simulink model "WT_MPPT_SCOPES_FINAL_v3"  (R2025a)
settings: Solver=ode4  StartTime=0.0  StopTime=11  FixedStep=0.1  RelTol=1e-3
settings Model: Creator=hero  LastModifiedBy=hero

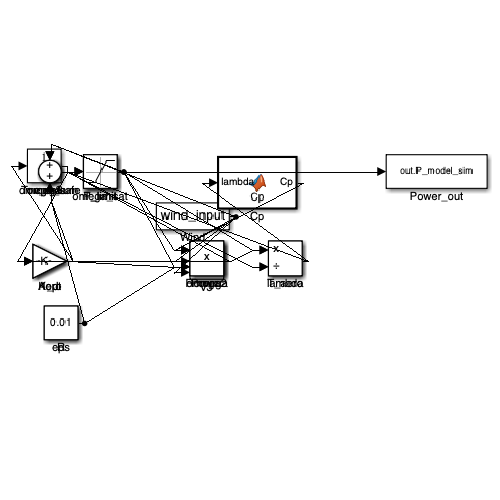
[thumbnail: Simulink's stored preview of the top-level diagram]
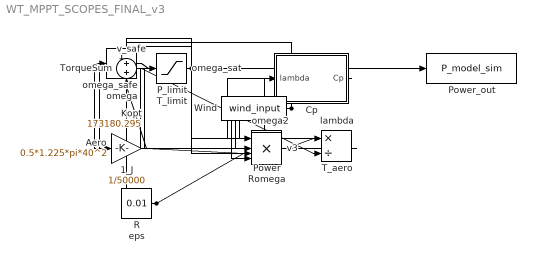
== system WT_MPPT_SCOPES_FINAL_v3 ==
  1_J : Gain  Gain=1/50000
  Aero : Gain  Gain=0.5*1.225*pi*40^2
  Cp : MATLAB Function  TreatAsAtomicUnit=on
  Kopt : Gain  Gain=173180.295
  P_limit : Saturate  UpperLimit=652.7945  LowerLimit=0
  Power : Product
  Power_out : ToWorkspace  VariableName=P_model_sim  SampleTime=-1
  R : Constant  Value=40
  Romega : Product
  T_aero : Product  Inputs=*/
  T_limit : Saturate  UpperLimit=1e6  LowerLimit=0
  TorqueSum : Sum  Inputs=+-
  Wind : FromWorkspace  VariableName=wind_input
  eps : Constant  Value=0.01
  lambda : Product  Inputs=*/
  omega : Integrator  InitialCondition=10
  omega2 : Product
  omega_safe : Sum
  omega_sat : Saturate  UpperLimit=100  LowerLimit=0.1
  v3 : Product  Inputs=3
  v_safe : Sum
  wires:
  omega/1 -> omega_sat/1
  omega_sat/1 -> Romega/1, omega_safe/1, omega2/1, omega2/2
  R/1 -> Romega/2
  Wind/1 -> v_safe/1, v3/1, v3/2, v3/3
  eps/1 -> v_safe/2, omega_safe/2
  Romega/1 -> lambda/1
  v_safe/1 -> lambda/2
  lambda/1 -> Cp/1(lambda)
  v3/1 -> Aero/1
  Aero/1 -> Power/2
  Cp/1(Cp) -> Power/1
  Power/1 -> P_limit/1
  P_limit/1 -> Power_out/1, T_aero/1
  omega_safe/1 -> T_aero/2
  T_aero/1 -> T_limit/1
  T_limit/1 -> TorqueSum/1
  omega2/1 -> Kopt/1
  Kopt/1 -> TorqueSum/2
  TorqueSum/1 -> 1_J/1
  1_J/1 -> omega/1

== matlab function WT_MPPT_SCOPES_FINAL_v3/Cp ==
  data: lambda input; Cp output
function Cp = Cp(lambda)
lambda = max(lambda,0.1);
lambda = min(lambda,12);
Cp = 0.22*((116./lambda)-5).*exp(-12.5./lambda);
Cp = max(min(Cp,0.5),0);
end
